simulink model "monofasikos_ask5_4xoritiko_monofasikos"  (R2021a)
settings: Solver=ode23tb  StartTime=0.0  StopTime=3  MaxStep=1e-5  RelTol=1e-3
undefined symbols (not defined in the file): L, R_vals
libraries: spsRMSLib x7, spsCurrentMeasurementLib x4, spsPowerLib x2, spsSeriesRLCBranchLib x2, spsVoltageMeasurementLib x2, spsControlledVoltageSourceLib x1, simulink x1, spsSaturableTransformerLib x1, spspowerguiLib x1
settings Model: Creator=epape  LastModifiedBy=epape

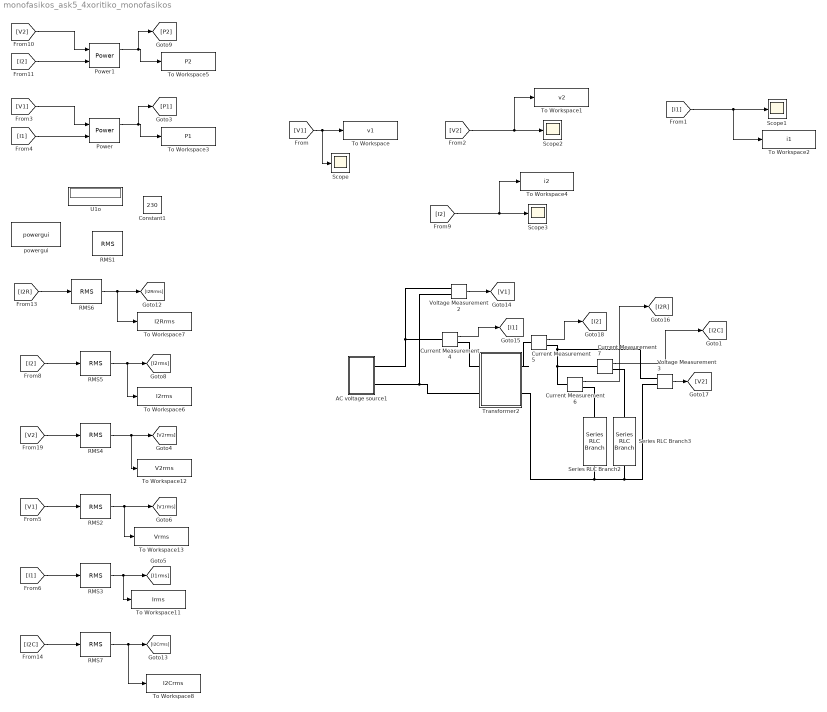
== system monofasikos_ask5_4xoritiko_monofasikos ==
  AC voltage source1 : Subsystem  mask{Vrms=230}
  Constant1 : Constant  Value=230
  Current Measurement{4..7} (4 alike) : spsCurrentMeasurementLib/Current Measurement  PhasorSimulation=off  OutputType=Complex  PSBequivalent=0
  Power : spsPowerLib/Power  Freq=50  Vinit=[0, 0]  Iinit=[0, 0]  Ts=1e-5
      settings: SourceProductBaseCode=PS
  Power1 : spsPowerLib/Power  Freq=50  Vinit=[0, 0]  Iinit=[0, 0]  Ts=1e-5
      settings: SourceProductBaseCode=PS
  RMS{1..7} (7 alike) : spsRMSLib/RMS  TrueRMS=on  Freq=50  RMSInit=0  Ts=0
  Scope{,1..3} (4 alike) : Scope
  Series RLC Branch2 : spsSeriesRLCBranchLib/Series RLC Branch  LConnTagsString=__new0  RConnTagsString=__new0  BranchType=R  Resistance=3.7  Inductance=1e-3  SetiL0=off  InitialCurrent=0  Capacitance=1e-6  Setx0=off  InitialVoltage=0  Measurements=None
  Series RLC Branch3 : spsSeriesRLCBranchLib/Series RLC Branch  LConnTagsString=__new0  RConnTagsString=__new0  BranchType=C  Resistance=R_vals(13)  Inductance=L  SetiL0=on  InitialCurrent=0  Capacitance=1.3739e-4  Setx0=on  InitialVoltage=0  Measurements=None
  To Workspace : ToWorkspace  VariableName=v1  SaveFormat=Timeseries  SampleTime=1e-5
  To Workspace1 : ToWorkspace  VariableName=v2  SaveFormat=Timeseries  SampleTime=1e-5
  To Workspace11 : ToWorkspace  VariableName=Irms  SaveFormat=Timeseries  SampleTime=1e-5
  To Workspace12 : ToWorkspace  VariableName=V2rms  SaveFormat=Timeseries  SampleTime=1e-5
  To Workspace13 : ToWorkspace  VariableName=Vrms  SaveFormat=Timeseries  SampleTime=1e-5
  To Workspace2 : ToWorkspace  VariableName=i1  SaveFormat=Timeseries  SampleTime=1e-5
  To Workspace3 : ToWorkspace  VariableName=P1  SaveFormat=Timeseries  SampleTime=1e-5
  To Workspace4 : ToWorkspace  VariableName=i2  SaveFormat=Timeseries  SampleTime=1e-5
  To Workspace5 : ToWorkspace  VariableName=P2  SaveFormat=Timeseries  SampleTime=1e-5
  To Workspace6 : ToWorkspace  VariableName=I2rms  SaveFormat=Timeseries  SampleTime=1e-5
  To Workspace7 : ToWorkspace  VariableName=I2Rrms  SaveFormat=Timeseries  SampleTime=1e-5
  To Workspace8 : ToWorkspace  VariableName=I2Crms  SaveFormat=Timeseries  SampleTime=1e-5
  Transformer2 : Subsystem  mask{PN=4, U1N=230, U2N=115}
      mask prompts: PN "PN (kVA)"; U1N "U1N (V)"; U2N "U2N (V)"
  U1o : Display
  Voltage Measurement2 : spsVoltageMeasurementLib/Voltage Measurement  PhasorSimulation=off  OutputType=Complex  PSBequivalent=0
  Voltage Measurement3 : spsVoltageMeasurementLib/Voltage Measurement  PhasorSimulation=off  OutputType=Complex  PSBequivalent=0
  powergui : spspowerguiLib/powergui  Priority=1  SimulationMode=Continuous  SampleTime=50e-6  frequency=60  Iterations=50  frequencyindice=0  Pbase=100e6  ErrMax=1e-4  UnitsV=kV  UnitsW=MW  buscounter=0  FunctionMessages=off  echomessages=off  EnableUseOfTLC=off  CurrentSourceSwitches=off  DisableSnubberDevices=off  DisableRonSwitches=off  DisableVfSwitches=off  DisplayEquations=off  AutomaticDiscreteSolvers=off  SolverType=Tustin/Backward Euler (TBE)  Interpol=off  ExternalGateDelay=off  methode=off  Ts=100  x0status=blocks  SPID=on  SwTol=0  HookPort=off  NonlinearTolerance=1e-4  nMaxIteration=100  ContinueOnMaxIteration=off  RestoreLinks=warning  ResistiveCurrentMeasurement=off  Frange=[0:2:500]  Ylog=off  Xlog=on  ShowGrid=off  save=off  variable=ZData  structure=0  ZoomFFT=off  StartTime=0.0  cycles=1  DisplayStyle=1  fundamental=60  FreqAxis=off  MaxFrequency=1000  frequencyindicesteady=1  RmsSteady=1  display=off
  wires:
  [I2] -> Power1/2
  [I1] -> To Workspace2/1, Scope1/1
  [I1] -> Power/2
  Power/1 -> [P1], To Workspace3/1
  [I2] -> To Workspace4/1, Scope3/1
  [V1] -> Power/1
  [V2] -> Power1/1
  Power1/1 -> [P2], To Workspace5/1
  [V1] -> Scope/1, To Workspace/1
  [V2] -> To Workspace1/1, Scope2/1
  RMS3/1 -> To Workspace11/1, [I1rms]
  RMS4/1 -> To Workspace12/1, [V2rms]
  [I1] -> RMS3/1
  [V1] -> RMS2/1
  RMS2/1 -> To Workspace13/1, [V1rms]
  RMS6/1 -> To Workspace7/1, [I2Rrms]
  [V2] -> RMS4/1
  [I2C] -> RMS7/1
  RMS5/1 -> To Workspace6/1, [I2rms]
  RMS7/1 -> To Workspace8/1, [I2Crms]
  [I2R] -> RMS6/1
  [I2] -> RMS5/1
  Current Measurement5/1 -> [I2]
  Voltage Measurement3/1 -> [V2]
  Current Measurement4/1 -> [I1]
  Current Measurement6/1 -> [I2R]
  Current Measurement7/1 -> [I2C]
  Voltage Measurement2/1 -> [V1]
  connections:
  Series RLC Branch2/RConn1 -- Voltage Measurement3/LConn2 -- Series RLC Branch3/RConn1 -- Transformer2/RConn2
  Current Measurement4/LConn1 -- Voltage Measurement2/LConn1 -- AC voltage source1/RConn1
  Transformer2/LConn2 -- AC voltage source1/RConn2 -- Voltage Measurement2/LConn2
  Current Measurement7/LConn1 -- Current Measurement6/LConn1 -- Current Measurement5/RConn1 -- Voltage Measurement3/LConn1
  Transformer2/RConn1 -- Current Measurement5/LConn1
  Current Measurement7/RConn1 -- Series RLC Branch3/LConn1
  Transformer2/LConn1 -- Current Measurement4/RConn1
  Current Measurement6/RConn1 -- Series RLC Branch2/LConn1

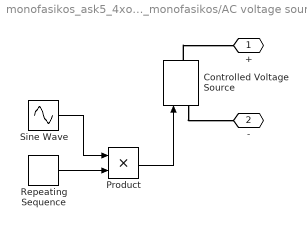
== system monofasikos_ask5_4xoritiko_monofasikos/AC voltage source1 ==
  Controlled Voltage Source : spsControlledVoltageSourceLib/Controlled Voltage Source  Initialize=on  Source_Type=AC  Amplitude=0  Phase=0  Frequency=50  Measurements=Voltage
  Product : Product
  Repeating Sequence : simulink/Sources/Repeating Sequence  rep_seq_t=[0 6]  rep_seq_y=[230 230]
  Sine Wave : Sin  Amplitude=sqrt(2)  Frequency=100*pi  SampleTime=0
  + : PMIOPort  Side=Right
  - : PMIOPort  Port=2  Side=Right
  wires:
  Product/1 -> Controlled Voltage Source/1
  Sine Wave/1 -> Product/1
  Repeating Sequence/1 -> Product/2
  connections:
  Controlled Voltage Source/LConn1 -- -/RConn1
  Controlled Voltage Source/RConn1 -- +/RConn1

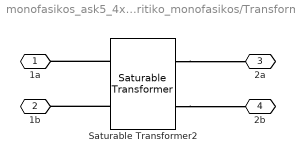
== system monofasikos_ask5_4xoritiko_monofasikos/Transformer2 ==
  Saturable Transformer2 : spsSaturableTransformerLib/Saturable Transformer  ThreeWindings=off  Hysteresis=off  DataFile='hysteresis.mat'  Measurements=Flux and excitation current ( Imag + IRm )  UNITS=pu  NominalPower=[4e3 50]  Winding1=[230 0.022273 0.015903]  Winding2=[122 0.024298 0.019083]  Winding3=[3.15e+05 0.00245 0.098001]  Saturation=[0 0;0.031714 0.76205;0.037813 0.86926;0.045538 0.94653;0.060175 1.0141;0.080911 1.0624;0.14637 1.159]  CoreLoss=35.539  BreakLoop=off  DiscreteSolver=Trapezoidal iterative  DataType=off  InitialFlux=0  TransfoNumber=1
      settings: SourceProductBaseCode=PS
  1a : PMIOPort  Side=Left
  1b : PMIOPort  Port=2  Side=Left
  2a : PMIOPort  Port=3  Side=Right
  2b : PMIOPort  Port=4  Side=Right
  connections:
  Saturable Transformer2/RConn2 -- 2b/RConn1
  Saturable Transformer2/LConn1 -- 1a/RConn1
  Saturable Transformer2/RConn1 -- 2a/RConn1
  Saturable Transformer2/LConn2 -- 1b/RConn1
